simulink model "using_labels_for_simplification"  (R2014b)
settings: Solver=ode23tb  StartTime=0.0  StopTime=1  RelTol=1e-3
libraries: powerlib_meascontrol x10, powerlib x6
settings Model: Creator=Amr Saleh  LastModifiedBy=Amr Saleh

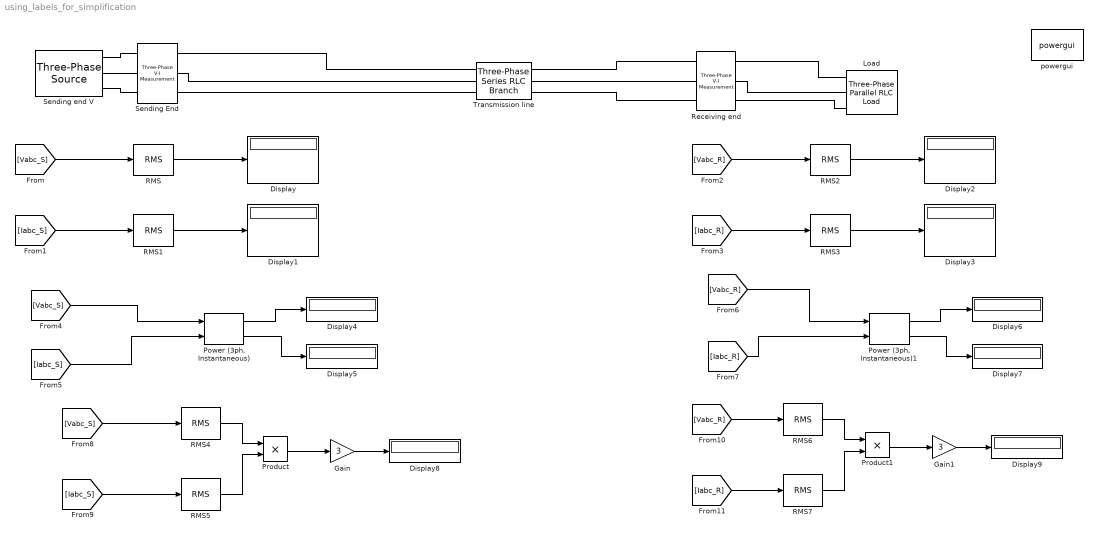
== system using_labels_for_simplification ==
  Display{,1..9} (10 alike) : Display
  Gain : Gain  Gain=3
  Gain1 : Gain  Gain=3
  Load : powerlib/Elements/Three-Phase Parallel RLC Load  LConnTagsString=A|B|C  Configuration=Y (grounded)  NominalVoltage=220e3  NominalFrequency=60  ActivePower=304.8e6  InductivePower=228.6e6  CapacitivePower=0  Measurements=None  LoadType=constant Z
  "Power (3ph, Instantaneous)" : powerlib_meascontrol/Measurements/Power (3ph, Instantaneous)
  "Power (3ph, Instantaneous)1" : powerlib_meascontrol/Measurements/Power (3ph, Instantaneous)
  Product : Product
  Product1 : Product
  RMS{,1..7} (8 alike) : powerlib_meascontrol/Measurements/RMS  TrueRMS=on  Freq=60  RMSInit=0  Ts=0
  Receiving end : powerlib/Measurements/Three-Phase V-I Measurement  VoltageMeasurement=phase-to-ground  SetLabelV=on  LabelV=Vabc_R  Vpu=off  VpuLL=off  CurrentMeasurement=yes  SetLabelI=on  LabelI=Iabc_R  Ipu=off  Pbase=100e6  Vbase=500e3  OutputType=Complex  PhasorSimulation=off  PSBequivalent=0
  Sending End : powerlib/Measurements/Three-Phase V-I Measurement  VoltageMeasurement=phase-to-ground  SetLabelV=on  LabelV=Vabc_S  Vpu=off  VpuLL=off  CurrentMeasurement=yes  SetLabelI=on  LabelI=Iabc_S  Ipu=off  Pbase=100e6  Vbase=500e3  OutputType=Complex  PhasorSimulation=off  PSBequivalent=0
  Sending end V : powerlib/Electrical Sources/Three-Phase Source  Voltage=250e3  PhaseAngle=0  Frequency=60  InternalConnection=Yg  SpecifyImpedance=off  Resistance=0  Inductance=0  ShortCircuitLevel=100e6  BaseVoltage=250e3  XRratio=7  BusType=swing  Pref=0  Qref=0  Qmin=-inf  Qmax=inf
  Transmission line : powerlib/Elements/Three-Phase Series RLC Branch  LConnTagsString=A|B|C  RConnTagsString=A|B|C  BranchType=RL  Resistance=6  Inductance=0.053052  Capacitance=1e-6  Measurements=None
  powergui : powerlib/powergui  Priority=1  SimulationMode=Continuous  SolverType=Tustin/Backward Euler (TBE)  SampleTime=50e-6  frequency=60  SPID=off  DisableSnubberDevices=off  DisableRonSwitches=off  DisableVfSwitches=off  SwTol=0  DisplayEquations=off  Interpol=off  methode=off  Ts=100  frequencyindice=60  Pbase=100e6  ErrMax=1e-4  Iterations=50  UnitsV=kV  UnitsW=MW  FunctionMessages=off  echomessages=off  HookPort=off  EnableUseOfTLC=off  x0status=blocks  RestoreLinks=warning  ResistiveCurrentMeasurement=off  Frange=[0:2:500]  Ylog=off  Xlog=on  ShowGrid=off  save=off  variable=ZData  structure=0  ZoomFFT=off  StartTime=0.0  cycles=1  DisplayStyle=1  fundamental=60  FreqAxis=off  MaxFrequency=1000  frequencyindicesteady=1  RmsSteady=1  display=off
  wires:
  [Iabc_S] -> RMS1/1
  [Vabc_S] -> RMS/1
  RMS/1 -> Display/1
  RMS1/1 -> Display1/1
  [Iabc_R] -> RMS3/1
  [Vabc_R] -> RMS2/1
  RMS2/1 -> Display2/1
  RMS3/1 -> Display3/1
  [Vabc_S] -> "Power (3ph, Instantaneous)"/1
  [Iabc_S] -> "Power (3ph, Instantaneous)"/2
  "Power (3ph, Instantaneous)"/1 -> Display4/1
  "Power (3ph, Instantaneous)"/2 -> Display5/1
  [Vabc_R] -> "Power (3ph, Instantaneous)1"/1
  [Iabc_R] -> "Power (3ph, Instantaneous)1"/2
  "Power (3ph, Instantaneous)1"/1 -> Display6/1
  "Power (3ph, Instantaneous)1"/2 -> Display7/1
  [Iabc_S] -> RMS5/1
  [Vabc_S] -> RMS4/1
  RMS4/1 -> Product/1
  RMS5/1 -> Product/2
  Product/1 -> Gain/1
  Gain/1 -> Display8/1
  [Iabc_R] -> RMS7/1
  [Vabc_R] -> RMS6/1
  RMS6/1 -> Product1/1
  RMS7/1 -> Product1/2
  Product1/1 -> Gain1/1
  Gain1/1 -> Display9/1
  connections:
  Sending end V/RConn1 -- Sending End/LConn1
  Sending end V/RConn2 -- Sending End/LConn2
  Sending end V/RConn3 -- Sending End/LConn3
  Transmission line/LConn1 -- Sending End/RConn1
  Transmission line/LConn2 -- Sending End/RConn2
  Transmission line/LConn3 -- Sending End/RConn3
  Receiving end/LConn1 -- Transmission line/RConn1
  Transmission line/RConn2 -- Receiving end/LConn2
  Transmission line/RConn3 -- Receiving end/LConn3
  Load/LConn1 -- Receiving end/RConn1
  Receiving end/RConn2 -- Load/LConn2
  Receiving end/RConn3 -- Load/LConn3
